simulink model "onezonevav"  (R2020a)
settings: Solver=FixedStepAuto  StartTime=0.0  StopTime=Inf  FixedStep=0.001  RelTol=1e-3
PostLoadFcn:
  | if any(exist('dsrtsu_mdlpostloadfcn', 'file') ~= 0), dsrtsu_mdlpostloadfcn('Execute', bdroot); end
InitFcn:
  | , if any(exist('rtifpga_mdlclblib', 'file') ~= 0), rtifpga_mdlclblib('Init', bdroot); end,
  | , if any(exist('dsmpb_private', 'file') ~= 0), dsmpb_private('dsmpb_mdlclblib', 'Init', bdroot); end,
libraries: dsmpblib x4
(part 1 of 3)
PreSaveFcn:
  | , if any(exist('dsmpb_private', 'file') ~= 0), dsmpb_private('dsmpb_mdlclblib', 'PreSave', bdroot); end,
CloseFcn:
  | , if any(exist('dsmpb_private', 'file') ~= 0), dsmpb_private('dsmpb_mdlclblib', 'Close', bdroot); end,
settings Model: RTICANMMDATA=struct('GeneralSetupData',struct('modelroot','D:\github\dspace-modelica-example\simulink\onezonevav','generalsettings',struct('filesettings',struct('destfolder',struct('Name','RTICANMM_FILES','Check',1),'buildfolder',struct('Name','.','Check',1),'AbsDestfolder',struct('Name','D:\github\dspace-modelica-example\simulink\onezonevav\RTICANMM_FILES'),'AbsBuildfolder',struct('Name','D:\github\dspace-modelica-example\simulink\onezonevav'))),'options',struct('addpaths',1,'rmpaths',1,'addtrcexclusion',true,'cannavigator',struct('checkmonitoring',0),'show_usrtrc',0,'use_usrtrc',0),'advanced',struct('options',ones(1,100)),'MPSetup',{{}},'RTI',struct('Type','DSRT','Ver','4.3','Date','02-May-2020'),'modelname','','block','untitled'))  DSRTSU_INTERNAL_RTIFPGA=160  DSMPB_ID_DATA={'71',struct('BlockId','862b8eba-4ab3-43e7-b955-ed32e3c107b3','SignalIds',{{'0ab8ee6c-7225-4ae8-94b1-2bf8a734a5aa'}}),'72',struct('BlockId','21139df6-93a0-414b-acd4-0a0addc88d9e','SignalIds',{{'81ce4164-1edd-44c7-a8f7-6a102065b527'}}),'73',struct('BlockId','cea0ac9a-86da-4945-a87c-4e9454283ce2','SignalIds',{{'f9a08468-eee7-4e09-b978-54f2c291118b'}}),'74',struct('BlockId','56948961-24e2-4f14-b37b-3d40fb51f202','SignalIds',{{'c42dede7-5ff3-4bd8-932f-075d532eb886'}})}  Creator=yangyang.fu  LastModifiedBy=yangyang.fu
settings OptimizationCC: BlockReduction=off  ConditionallyExecuteInputs=off  OptimizeBlockIOStorage=off  BufferReuse=off
settings DebuggingCC: TasksWithSamePriorityMsg=none
settings HardwareCC: ProdBitPerPointer=32  ProdBitPerSizeT=32  ProdBitPerPtrDiffT=32  ProdLargestAtomicInteger=Integer  ProdWordSize=32  ProdLongLongMode=on  ProdHWDeviceType=Custom Processor->Custom
settings ModelReferenceCC: EnableParallelModelReferenceBuilds=on
settings SFSimCC: MATLABDynamicMemAlloc=off
settings RTWCC: Description=dSPACE Run-Time Target (for VEOS on Windows and ConfigurationDesk)  SystemTargetFile=dsrt.tlc  GenCodeOnly=on  MakeCommand=make_dsrt  TemplateMakefile=dsrt_default_tmf  RTWVerbose=off  CustomInclude="\"C:\\Program Files\\Dymola 2021\\Source\""
settings STFCustomTargetCC: TargetLangStandard=C99 (ISO)  ParMdlRefBuildCompliant=on  SystemTargetFile=dsrt.tlc
settings GRTTargetCC: CompOptLevelCompliant=off  ConcurrentExecutionCompliant=off  CombineOutputUpdateFcns=off  MatFileLogging=off  CPPClassGenCompliant=off  UseToolchainInfoCompliant=off

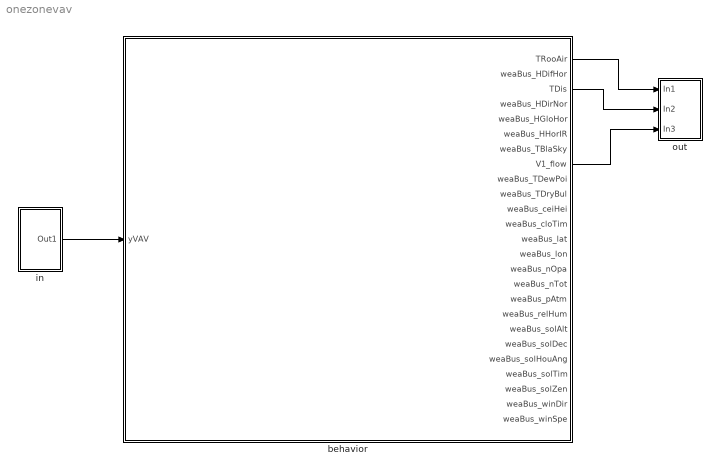
== system onezonevav ==
  behavior : Subsystem
  in : Subsystem
  out : Subsystem
  wires:
  behavior/1(TRooAir) -> out/1(In1)
  behavior/3(TDis) -> out/2(In2)
  behavior/8(V1_flow) -> out/3(In3)
  in/1(Out1) -> behavior/1(yVAV)

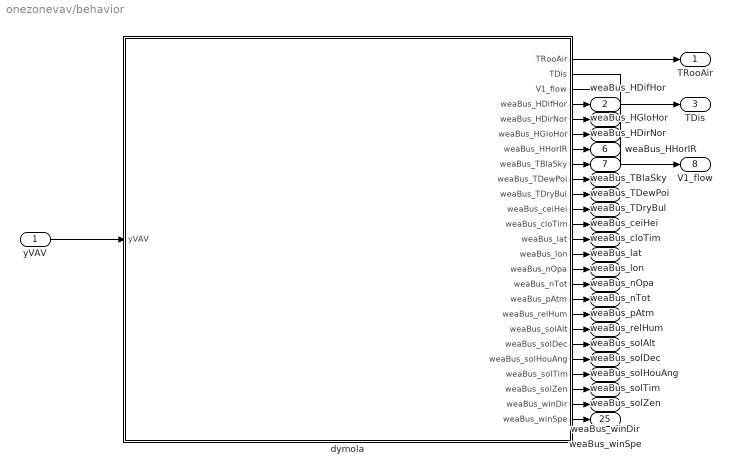
== system onezonevav/behavior ==
  yVAV : Inport
  dymola : Subsystem  Tag=08-Nov-2021 17:14:02#4218
      mask help:
      | Dymola block.
      | A dymola block allows acausal physical modeling.
      | See Dymola manual for usage.
      settings: CopyFcn=newDymolaGui('08-Nov-2021 17:14:02#4218','Copy');  DeleteFcn=if exist('newDymolaGui') newDymolaGui('onezonevav/behavior/dymola','Delete'); end;  NameChangeFcn=newDymolaGui('08-Nov-2021 17:14:02#4218','Copy');  OpenFcn=newDymolaGui('onezonevav/behavior/dymola','Init');
      mask Display: image(reshape([1;1;1;1;1;1;1;1;1;1;1;1;1;1;1;1;1;1;1;1;1;1;0;0;0;0;0;0;0;0;0;0;1;1;1;1;1;1;1;1;0;1;1;1;1;1;1;1;1;0;1;1;1;1;1;0;0;0;0;0;0;0;1;1;0;0;0;0;0;0;0;1;1;0;0;0;0;0;0;0;1;1;0;0;0;0;0;0;0;1;1;0;0;0;0;0;0;0;1;1;0;0;0;0;0;0;0;1;1;0;0;0;0;0;0;0;1;1;0;0;0;0;0;0;0;1;1;0;0;0;0;0;0;0;1;1;0;0;0;0;0;0;0;1;1;0;0;0;0;0;0;0;1;1;0;0;0;0;0;0;0;1;1;0;0;0;0;0;0;0;1;1;0;0;0;0;0;0;0;1;1;0;0;0;0;0;0;0;1;1;0;0;0;0;0;0;0;1;1;0;0;0;0;0;0;0;1;1;0;0;0;0;0;0;0;1;1;0;0;0;0;0;0;0;1;1;0;0;0;0;0;0;0;1;1;0;0;0;0;0;0;0;1;1;0;0;0;0;0;0;0;1;1;0;0;0;0;0;0;0;1;1;0;0;0;0;0;0;0;1;1;1;1;1;0;1;1;1;1;1;1;1;1;0;1;1;1;1;1;1;1;1;0;0;0;0;0;0;0;0;0;0;1;1;1;1;1;1;1;1;1;1;1;1;1;1;1;1;1;1;1;1;1;1;1;1;1;1;1;1;1;1;1;1;1;1;1;1;1;1;1;1;1;1;1;1;0;0;0;0;0;0;0;0;0;0;1;1;1;1;1;1;1;1;0;1;1;1;1;1;1;1;1;0;1;1;1;1;1;0;0;0;0;0;0;0;1;1;0;0;0;0;0;0;0;1;1;0;0;0;0;0;0;0;1;1;0;0;0;0;0;0;0;1;1;0;0;0;0;0;0;0;1;1;0;0;0;0;0;0;0;1;1;0;0;0;0;0;0;0;1;1;0;0;0;0;0;0;0;1;1;0;0;0;0;0;0;0;1;1;0;0;0;0;0;0;0;1;1;0;0;0;0;0;0;0;1;1;0;0;0;0;0;0;0;1;1;0;0;0;0;0;0;0;1;1;0;0;0;0;0;0;0;1;1;0;0;0;0;0;0;0;1;1;0;0;0;0;0;0;0;1;1;0;0;0;0;0;0;0;1;1;0;0;0;0;0;0;0;1;1;0;0;0;0;0;0;0;1;1;0;0;0;0;0;0;0;1;1;0;0;0;0;0;0;0;1;1;0;0;0;0;0;0;0;1;1;0;0;0;0;0;0;0;1;1;0;0;0;0;0;0;0;1;1;1;1;1;0;1;1;1;1;1;1;1;1;0;1;1;1;1;1;1;1;1;0;0;0;0;0;0;0;0;0;0;1;1;1;1;1;1;1;1;1;1;1;1;1;1;1;1;1;1;1;1;1;1;1;1;1;1;1;1;1;1;1;1;1;1;1;1;1;1;1;1;1;1;1;1;0;0;0;0;0;0;0;0;0;0;1;1;1;1;1;1;1;1;0;1;1;1;1;1;1;1;1;0;1;1;1;1;1;0;0;0;0;0;0;0;1;1;0;0;0;0;0;0;0;1;1;0;1;1;1;1;1;0;1;1;0;1;1;1;1;1;0;1;1;0;1;1;1;1;1;0;1;1;0;1;1;1;1;1;0;1;1;0;1;1;1;1;1;0;1;1;0;1;1;1;1;1;0;1;1;0;1;1;1;1;1;0;1;1;0;1;1;1;1;1;0;1;1;0;1;1;1;1;1;0;1;1;0;1;1;1;1;1;0;1;1;0;1;1;1;1;1;0;1;1;0;1;1;1;1;1;0;1;1;0;1;1;1;1;1;0;1;1;0;1;1;1;1;1;0;1;1;0;1;1;1;1;1;0;1;1;0;1;1;1;1;1;0;1;1;0;1;1;1;1;1;0;1;1;0;1;1;1;1;1;0;1;1;0;1;1;1;1;1;0;1;1;0;1;1;1;1;1;0;1;1;0;0;0;0;0;0;0;1;1;0;0;0;0;0;0;0;1;1;1;1;1;0;1;1;1;1;1;1;1;1;0;1;1;1;1;1;1;1;1;0;0;0;0;0;0;0;0;0;0;1;1;1;1;1;1;1;1;1;1;1;1;1;1;1;1;1;1;1;1;1;1],18,18,3),[.2,.2,.6,.6])
  TRooAir : Outport
  weaBus_HDifHor : Outport  Port=2
  TDis : Outport  Port=3
  weaBus_HDirNor : Outport  Port=4
  weaBus_HGloHor : Outport  Port=5
  weaBus_HHorIR : Outport  Port=6
  weaBus_TBlaSky : Outport  Port=7
  V1_flow : Outport  Port=8
  weaBus_TDewPoi : Outport  Port=9
  weaBus_TDryBul : Outport  Port=10
  weaBus_ceiHei : Outport  Port=11
  weaBus_cloTim : Outport  Port=12
  weaBus_lat : Outport  Port=13
  weaBus_lon : Outport  Port=14
  weaBus_nOpa : Outport  Port=15
  weaBus_nTot : Outport  Port=16
  weaBus_pAtm : Outport  Port=17
  weaBus_relHum : Outport  Port=18
  weaBus_solAlt : Outport  Port=19
  weaBus_solDec : Outport  Port=20
  weaBus_solHouAng : Outport  Port=21
  weaBus_solTim : Outport  Port=22
  weaBus_solZen : Outport  Port=23
  weaBus_winDir : Outport  Port=24
  weaBus_winSpe : Outport  Port=25
  wires:
  dymola/19(weaBus_solAlt) -> weaBus_solAlt/1
  dymola/7(weaBus_HHorIR) -> weaBus_HHorIR/1
  dymola/4(weaBus_HDifHor) -> weaBus_HDifHor/1
  dymola/3(V1_flow) -> V1_flow/1
  dymola/9(weaBus_TDewPoi) -> weaBus_TDewPoi/1
  dymola/10(weaBus_TDryBul) -> weaBus_TDryBul/1
  dymola/8(weaBus_TBlaSky) -> weaBus_TBlaSky/1
  dymola/21(weaBus_solHouAng) -> weaBus_solHouAng/1
  dymola/5(weaBus_HDirNor) -> weaBus_HDirNor/1
  dymola/20(weaBus_solDec) -> weaBus_solDec/1
  dymola/6(weaBus_HGloHor) -> weaBus_HGloHor/1
  yVAV/1 -> dymola/1(yVAV)
  dymola/24(weaBus_winDir) -> weaBus_winDir/1
  dymola/11(weaBus_ceiHei) -> weaBus_ceiHei/1
  dymola/12(weaBus_cloTim) -> weaBus_cloTim/1
  dymola/13(weaBus_lat) -> weaBus_lat/1
  dymola/16(weaBus_nTot) -> weaBus_nTot/1
  dymola/1(TRooAir) -> TRooAir/1
  dymola/17(weaBus_pAtm) -> weaBus_pAtm/1
  dymola/2(TDis) -> TDis/1
  dymola/15(weaBus_nOpa) -> weaBus_nOpa/1
  dymola/14(weaBus_lon) -> weaBus_lon/1
  dymola/18(weaBus_relHum) -> weaBus_relHum/1
  dymola/22(weaBus_solTim) -> weaBus_solTim/1
  dymola/23(weaBus_solZen) -> weaBus_solZen/1
  dymola/25(weaBus_winSpe) -> weaBus_winSpe/1

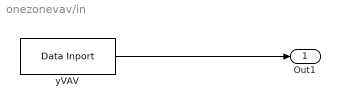
== system onezonevav/in ==
  yVAV : dsmpblib/Data Inport  Priority=10000
      settings: SourceProductName=dSPACE Model Interface Blockset
  Out1 : Outport
  wires:
  yVAV/1 -> Out1/1

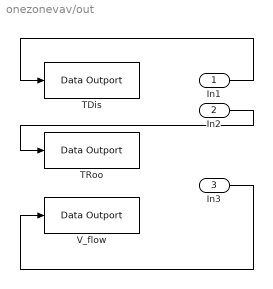
== system onezonevav/out ==
  In1 : Inport
  In2 : Inport  Port=2
  In3 : Inport  Port=3
  TDis : dsmpblib/Data Outport  Priority=-10000
      settings: SourceProductName=dSPACE Model Interface Blockset
  TRoo : dsmpblib/Data Outport  Priority=-10000
      settings: SourceProductName=dSPACE Model Interface Blockset
  V_flow : dsmpblib/Data Outport  Priority=-10000
      settings: SourceProductName=dSPACE Model Interface Blockset
  wires:
  In1/1 -> TDis/1
  In2/1 -> TRoo/1
  In3/1 -> V_flow/1
